simulink model "pdm_pcm"  (R2017b)
settings: Solver=ode5  StartTime=0.0  StopTime=t_duration  RelTol=1e-3
values from neighbouring files (symbols this model uses):
  fs = 8e3    (= 8000)    [PCM_PDM_PCM.m]
undefined symbols (not defined in the file or in its folder): d_fac, f_sr, N
libraries: dspmlti4 x3
settings Model: Creator=Dmitr  LastModifiedBy=Dmitr
settings OptimizationCC: RollThreshold=2

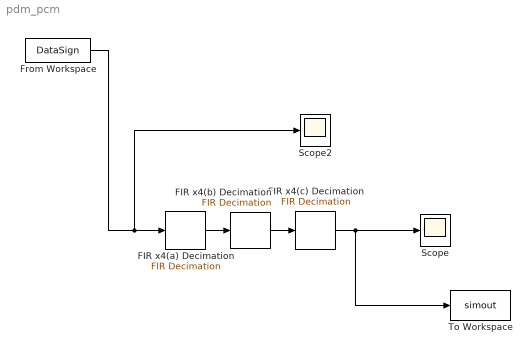
== system pdm_pcm ==
  FIR x4(a) Decimation : dspmlti4/FIR Decimation  FilterSource=Dialog parameters  h=fir1(N ,f_sr)  D=d_fac  filtStruct=Direct form  FilterObject=Hm_firdecim  framing=Allow multirate processing  inputOffset=0  outputBufInitCond=0  roundingMode=Floor  overflowMode=off  firstCoeffDataTypeStr=Inherit: Same word length as input  firstCoeffMin=[]  firstCoeffMax=[]  firstCoeffLastDataTypeStr=Inherit: Same word length as input  accumDataTypeStr=Inherit: Same as product output  accumLastDataTypeStr=Inherit: Same as product output  outputMin=[]  outputMax=[]
  FIR x4(b) Decimation : dspmlti4/FIR Decimation  FilterSource=Dialog parameters  h=fir1(N ,f_sr)  D=d_fac  filtStruct=Direct form  FilterObject=Hm_firdecim  framing=Allow multirate processing  inputOffset=0  outputBufInitCond=0  roundingMode=Floor  overflowMode=off  firstCoeffDataTypeStr=Inherit: Same word length as input  firstCoeffMin=[]  firstCoeffMax=[]  firstCoeffLastDataTypeStr=Inherit: Same word length as input  accumDataTypeStr=Inherit: Same as product output  accumLastDataTypeStr=Inherit: Same as product output  outputMin=[]  outputMax=[]
  FIR x4(c) Decimation : dspmlti4/FIR Decimation  FilterSource=Dialog parameters  h=fir1(N, f_sr)  D=d_fac  filtStruct=Direct form  FilterObject=Hm_firdecim  framing=Allow multirate processing  inputOffset=0  outputBufInitCond=0  roundingMode=Floor  overflowMode=off  firstCoeffDataTypeStr=Inherit: Same word length as input  firstCoeffMin=[]  firstCoeffMax=[]  firstCoeffLastDataTypeStr=Inherit: Same word length as input  accumDataTypeStr=Inherit: Same as product output  accumLastDataTypeStr=Inherit: Same as product output  outputMin=[]  outputMax=[]
  From Workspace : FromWorkspace  VariableName=DataSign  SampleTime=1/fs
  Scope : Scope
  Scope2 : Scope
  To Workspace : ToWorkspace  VariableName=simout  SampleTime=64/fs
      settings: Save2DSignal=2-D array (concatenate along first dimension)
  wires:
  From Workspace/1 -> Scope2/1, FIR x4(a) Decimation/1
  FIR x4(a) Decimation/1 -> FIR x4(b) Decimation/1
  FIR x4(b) Decimation/1 -> FIR x4(c) Decimation/1
  FIR x4(c) Decimation/1 -> To Workspace/1, Scope/1
